simulink model "s4stp"  (Simulink 2.00)
settings: Solver=ode15s  StartTime=0.0  StopTime=1.2  MaxStep=0.0005  RelTol=1e-6  AbsTol=1e-6
values from neighbouring files (symbols this model uses):
  Domega = 0    [P1HP.M]    (also in PSPH.M)
  H = J*wbm*wbm/(2*Sb)    (= 2.36870505626)    [P1HP.M]    (also in PSPH.M = 1.39074103839)
  Psidso = 0    [M1.M]    (also in M4.M; M4STP.M; M5.M)
  Psipdro = 0    [M1.M]    (also in M4.M; M4STP.M; M5.M; M6.M)
  Psipqro = 0    [M1.M]    (also in M4.M = Vm; M4STP.M = Vm; M5.M; M6.M)
  Psiqso = 0    [M1.M]    (also in M4.M = Vm; M4STP.M = Vm; M5.M; M6.M)
  rpr = 1.99    [P1HP.M]    (also in PSPH.M = 4.12)
  rs = 3.35    [P1HP.M]
  Tb = Sb/wbm    (= 3.9788735773)    [P1HP.M]    (also in PSPH.M = 0.989413229555)
  Tfactor = (3*P)/(4*wb)    (= 0.00795774715459)    [P1HP.M]    (also in PSPH.M = 0.00530516476973)
  wb = 2*pi*frated    (= 376.991118431)    [P1HP.M]    (also in PSPH.M)
  we = wb    (= 376.991118431)    [P1HP.M]    (also in PSPH.M)
  wrbywbo = 0    [M1.M]    (also in M4.M = 1; M4STP.M = 1; M5.M; M6.M)
  xls = 6.94e-3*wb    (= 2.61631836191)    [P1HP.M]
  xM = 1/(1/xm + 1/xls + 1/xplr)    (= 1.2810101836)    [P1HP.M]
  xplr = xls    (= 2.61631836191)    [P1HP.M]    (also in PSPH.M = 2.12)
settings Model: SaveTime=off  SaveOutput=off  ConsistencyChecking=off

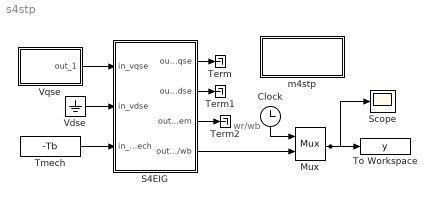
== system s4stp ==
  note: wr/wb
  Clock : Clock
      settings: Orientation=down  DeleteFcn=simclock BlockIsBeingDestroyed  PostSaveFcn=simclock Save
  m4stp : Subsystem
      settings: OpenFcn=m4stp
      mask Type: Masked block of m4stp.m
      mask Help: Uses m4stp.m to initialize and plot
      mask Display: disp('Initialize\nand plot')
  Mux : Mux  Inputs=2
  Scope : Scope
      settings: TickLabels=on  TimeRange=1.200000  YMin=-2.000000  YMax=2.000000  SaveToWorkspace=off  SaveName=ScopeData
  Term : Terminator
  Term1 : Terminator
  Term2 : Terminator
  Tmech : Constant  Value=-Tb
  To Workspace : ToWorkspace  VariableName=y  SampleTime=0
      settings: Buffer=500
  Vdse : Ground
  Vqse : Subsystem  mask(Repeating table){@1=[0 1 1 1.2], @2=[Vm Vm Vm+1 Vm+1]}
      mask prompts: @1 "Time values:"; @2 "Output values:"
      mask help:
      | Repeating table.
      | Enter values of time and output for first cycle.
      mask init:
      | period = max(@1); t = @1; y = @2;
      mask Help: Repeats cycle given in table. Time values should be monotonically increasing.
      mask Display: plot([t,t+period,t+2*period],[y,y,y])
  S4EIG : Subsystem
  wires:
  S4EIG/3(out_Tem) -> Term2/1
  Mux/1 -> Scope/1, To Workspace/1
  S4EIG/4(out_wr/wb) -> Mux/2
  Clock/1 -> Mux/1
  S4EIG/2(out_idse) -> Term1/1
  S4EIG/1(out_iqse) -> Term/1
  Tmech/1 -> S4EIG/3(in_Tmech)
  Vqse/1(out_1) -> S4EIG/1(in_vqse)
  Vdse/1 -> S4EIG/2(in_vdse)

== system s4stp/m4stp ==
  note: This masked block uses m4stp.m
      | to initialize the s4stp.m with
      | machine parameters and plot the simulated
      | results.

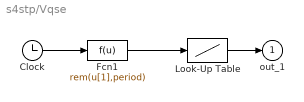
== system s4stp/Vqse ==
  Clock : Clock
      settings: DeleteFcn=simclock BlockIsBeingDestroyed  PostSaveFcn=simclock Save
  Fcn1 : Fcn  Expr=rem(u[1],period)
  Look-Up Table : Lookup  InputValues=t  OutputValues=y
  out_1 : Outport  Port=1  InitialOutput=0
  wires:
  Fcn1/1 -> Look-Up Table/1
  Clock/1 -> Fcn1/1
  Look-Up Table/1 -> out_1/1

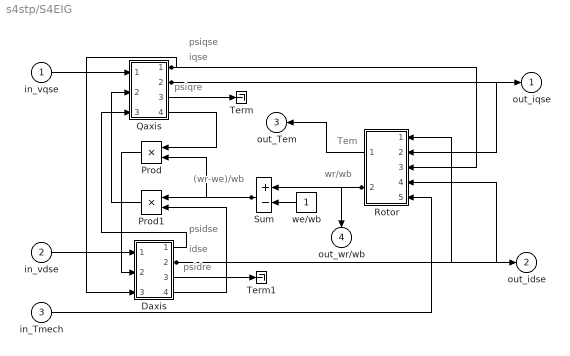
== system s4stp/S4EIG ==
  note: (wr-we)/wb
  note: iqse
  note: psiqse
  note: wr/wb
  note: Tem
  note: idse
  note: psidre
  note: psiqre
  note: psidse
  in_vqse : Inport  Port=1  PortWidth=-1  SampleTime=-1
  in_vdse : Inport  Port=2  PortWidth=-1  SampleTime=-1
  in_Tmech : Inport  Port=3  PortWidth=-1  SampleTime=-1
  Daxis : Subsystem
  Prod : Product  Orientation=left  Inputs=2
  Prod1 : Product  Orientation=left  Inputs=2
  Qaxis : Subsystem
  Rotor : Subsystem  Orientation=left
  Sum : Sum  Orientation=left  Inputs=+-
  Term : Terminator
  Term1 : Terminator
  we/wb : Constant  Orientation=left  Value=1
  out_iqse : Outport  Port=1  InitialOutput=0
  out_idse : Outport  Port=2  InitialOutput=0
  out_Tem : Outport  Orientation=left  Port=3  InitialOutput=0
  out_wr/wb : Outport  Orientation=down  Port=4  InitialOutput=0
  wires:
  Daxis/3(out_idr') -> Term1/1
  Qaxis/3(out_iqr') -> Term/1
  in_Tmech/1 -> Rotor/5(in_Tmech)
  Daxis/1(out_psids) -> Qaxis/3(in_psids)
  in_vdse/1 -> Daxis/1(in_vds)
  Rotor/2(out_wr/wb) -> out_wr/wb/1, Sum/1
  Rotor/1(out_Tem) -> out_Tem/1
  Qaxis/2(out_iqs) -> out_iqse/1, Rotor/2(in_iqse)
  in_vqse/1 -> Qaxis/1(in_vqs)
  Daxis/4(out_psidr') -> Prod1/2
  Qaxis/4(out_psiqr') -> Prod/1
  Daxis/2(out_ids) -> out_idse/1, Rotor/1(in_psidse), Rotor/4(in_idse)
  Prod/1 -> Daxis/2(in_(wr/wb)*psiqr')
  Qaxis/1(out_psiqs) -> Rotor/3(in_psiqse), Daxis/3(in_psiqs)
  Prod1/1 -> Qaxis/2((wr-we)*psidr'/wb)
  we/wb/1 -> Sum/2
  Sum/1 -> Prod/2, Prod1/1

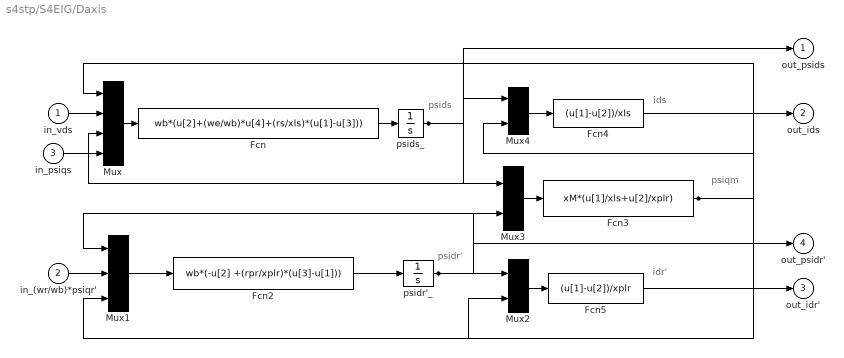
== system s4stp/S4EIG/Daxis ==
  note: ids
  note: psids
  note: psiqm
  note: idr'
  note: psidr'
  in_vds : Inport  Port=1  PortWidth=-1  SampleTime=-1
  in_(wr/wb)*psiqr' : Inport  Port=2  PortWidth=-1  SampleTime=-1
  in_psiqs : Inport  Port=3  PortWidth=-1  SampleTime=-1
  Fcn : Fcn  Expr=wb*(u[2]+(we/wb)*u[4]+(rs/xls)*(u[1]-u[3]))
  Fcn2 : Fcn  Expr=wb*(-u[2] +(rpr/xplr)*(u[3]-u[1]))
  Fcn3 : Fcn  Expr=xM*(u[1]/xls+u[2]/xplr)
  Fcn4 : Fcn  Expr=(u[1]-u[2])/xls
  Fcn5 : Fcn  Expr=(u[1]-u[2])/xplr
  Mux : Mux  Inputs=4
  Mux1 : Mux  Inputs=3
  Mux2 : Mux  Inputs=2
  Mux3 : Mux  Inputs=2
  Mux4 : Mux  Inputs=2
  psidr'_ : Integrator  ExternalReset=none  InitialConditionSource=internal  InitialCondition=Psipdro  LimitOutput=off  UpperSaturationLimit=inf  LowerSaturationLimit=-inf  ShowSaturationPort=off  ShowStatePort=off  AbsoluteTolerance=auto
  psids_ : Integrator  ExternalReset=none  InitialConditionSource=internal  InitialCondition=Psidso  LimitOutput=off  UpperSaturationLimit=inf  LowerSaturationLimit=-inf  ShowSaturationPort=off  ShowStatePort=off  AbsoluteTolerance=auto
  out_psids : Outport  Port=1  InitialOutput=0
  out_ids : Outport  Port=2  InitialOutput=0
  out_idr' : Outport  Port=3  InitialOutput=0
  out_psidr' : Outport  Port=4  InitialOutput=0
  wires:
  in_psiqs/1 -> Mux/4
  Fcn5/1 -> out_idr'/1
  in_(wr/wb)*psiqr'/1 -> Mux1/2
  in_vds/1 -> Mux/2
  Fcn4/1 -> out_ids/1
  Mux/1 -> Fcn/1
  Fcn/1 -> psids_/1
  Fcn2/1 -> psidr'_/1
  Mux3/1 -> Fcn3/1
  Mux4/1 -> Fcn4/1
  psids_/1 -> out_psids/1, Mux3/1, Mux4/1, Mux/3
  Fcn3/1 -> Mux4/2, Mux1/3, Mux/1, Mux2/2
  Mux1/1 -> Fcn2/1
  psidr'_/1 -> out_psidr'/1, Mux1/1, Mux3/2, Mux2/1
  Mux2/1 -> Fcn5/1

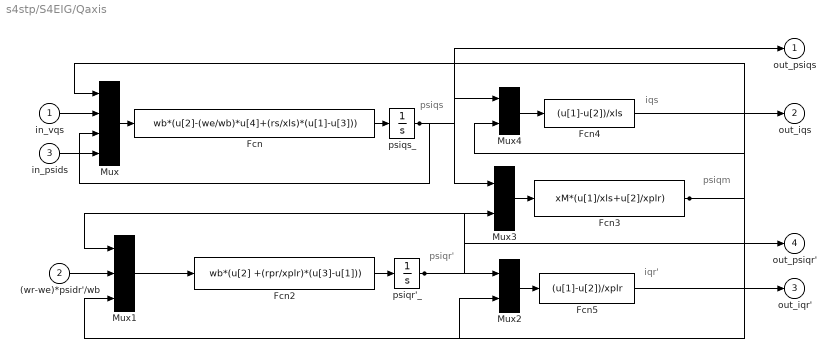
== system s4stp/S4EIG/Qaxis ==
  note: iqs
  note: psiqs
  note: psiqm
  note: iqr'
  note: psiqr'
  in_vqs : Inport  Port=1  PortWidth=-1  SampleTime=-1
  (wr-we)*psidr'/wb : Inport  Port=2  PortWidth=-1  SampleTime=-1
  in_psids : Inport  Port=3  PortWidth=-1  SampleTime=-1
  Fcn : Fcn  Expr=wb*(u[2]-(we/wb)*u[4]+(rs/xls)*(u[1]-u[3]))
  Fcn2 : Fcn  Expr=wb*(u[2] +(rpr/xplr)*(u[3]-u[1]))
  Fcn3 : Fcn  Expr=xM*(u[1]/xls+u[2]/xplr)
  Fcn4 : Fcn  Expr=(u[1]-u[2])/xls
  Fcn5 : Fcn  Expr=(u[1]-u[2])/xplr
  Mux : Mux  Inputs=4
  Mux1 : Mux  Inputs=3
  Mux2 : Mux  Inputs=2
  Mux3 : Mux  Inputs=2
  Mux4 : Mux  Inputs=2
  psiqr'_ : Integrator  ExternalReset=none  InitialConditionSource=internal  InitialCondition=Psipqro  LimitOutput=off  UpperSaturationLimit=inf  LowerSaturationLimit=-inf  ShowSaturationPort=off  ShowStatePort=off  AbsoluteTolerance=auto
  psiqs_ : Integrator  ExternalReset=none  InitialConditionSource=internal  InitialCondition=Psiqso  LimitOutput=off  UpperSaturationLimit=inf  LowerSaturationLimit=-inf  ShowSaturationPort=off  ShowStatePort=off  AbsoluteTolerance=auto
  out_psiqs : Outport  Port=1  InitialOutput=0
  out_iqs : Outport  Port=2  InitialOutput=0
  out_iqr' : Outport  Port=3  InitialOutput=0
  out_psiqr' : Outport  Port=4  InitialOutput=0
  wires:
  in_psids/1 -> Mux/4
  Fcn5/1 -> out_iqr'/1
  (wr-we)*psidr'/wb/1 -> Mux1/2
  in_vqs/1 -> Mux/2
  Fcn4/1 -> out_iqs/1
  Mux/1 -> Fcn/1
  Fcn/1 -> psiqs_/1
  Fcn2/1 -> psiqr'_/1
  Mux3/1 -> Fcn3/1
  Mux4/1 -> Fcn4/1
  psiqs_/1 -> out_psiqs/1, Mux3/1, Mux4/1, Mux/3
  Fcn3/1 -> Mux4/2, Mux1/3, Mux/1, Mux2/2
  Mux1/1 -> Fcn2/1
  psiqr'_/1 -> out_psiqr'/1, Mux1/1, Mux3/2, Mux2/1
  Mux2/1 -> Fcn5/1

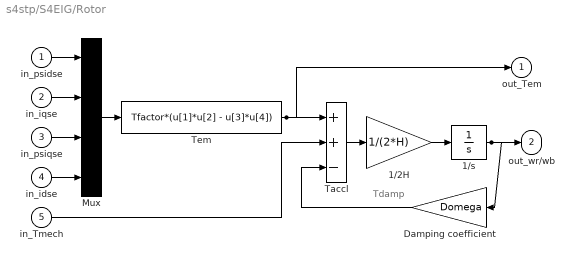
== system s4stp/S4EIG/Rotor ==
  note: Tdamp
  in_psidse : Inport  Port=1  PortWidth=-1  SampleTime=-1
  in_iqse : Inport  Port=2  PortWidth=-1  SampleTime=-1
  in_psiqse : Inport  Port=3  PortWidth=-1  SampleTime=-1
  in_idse : Inport  Port=4  PortWidth=-1  SampleTime=-1
  in_Tmech : Inport  Port=5  PortWidth=-1  SampleTime=-1
  1/2H : Gain  Gain=1/(2*H)
  1/s : Integrator  ExternalReset=none  InitialConditionSource=internal  InitialCondition=wrbywbo  LimitOutput=off  UpperSaturationLimit=inf  LowerSaturationLimit=-inf  ShowSaturationPort=off  ShowStatePort=off  AbsoluteTolerance=auto
  Damping coefficient : Gain  Orientation=left  Gain=Domega
  Mux : Mux  Inputs=4
  Taccl : Sum  Inputs=++-
  Tem : Fcn  Expr=Tfactor*(u[1]*u[2] - u[3]*u[4])
  out_Tem : Outport  Port=1  InitialOutput=0
  out_wr/wb : Outport  Port=2  InitialOutput=0
  wires:
  in_idse/1 -> Mux/4
  in_psiqse/1 -> Mux/3
  in_iqse/1 -> Mux/2
  in_psidse/1 -> Mux/1
  Mux/1 -> Tem/1
  1/s/1 -> out_wr/wb/1, Damping coefficient/1
  in_Tmech/1 -> Taccl/2
  Taccl/1 -> 1/2H/1
  1/2H/1 -> 1/s/1
  Tem/1 -> Taccl/1, out_Tem/1
  Damping coefficient/1 -> Taccl/3
